simulink model "amon_model"  (R2025b)
settings: Solver=VariableStepAuto  StartTime=0.0  StopTime=dt  RelTol=1e-3
undefined symbols (not defined in the file or in its folder): EDF_max, EDF_min, g, servo1_offset, servo2_offset, servo3_offset, servo4_offset, servo_max, servo_min, tau_edf, tau_servo
libraries: simulink x1
settings Model: Creator=titit  LastModifiedBy=titit

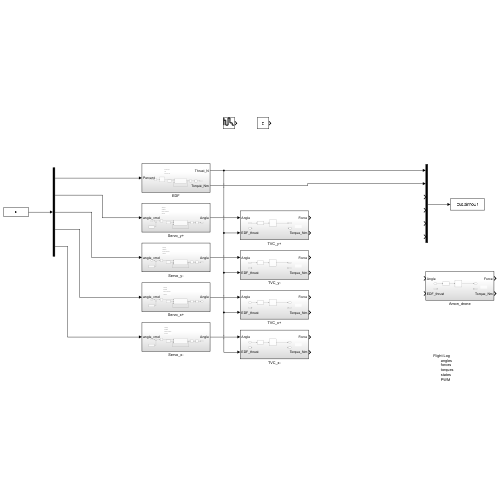
[thumbnail: Simulink's stored preview of the top-level diagram]
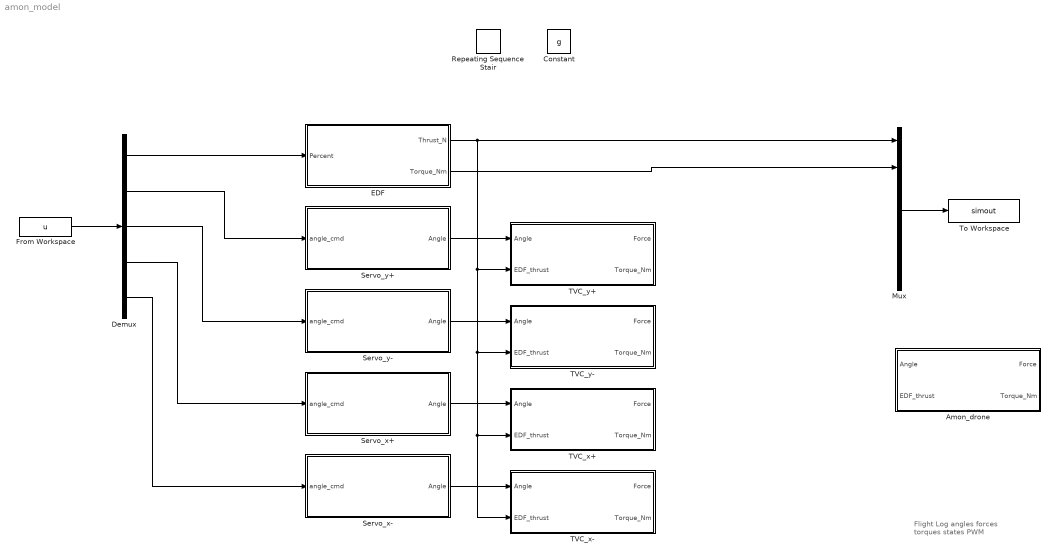
== system amon_model ==
  note: Flight Log
      | 	angles
      | 	forces
      | 	torques
      | 	states
      | 	PWM
  Amon_drone : Subsystem
  Constant : Constant  Value=g
  Demux : Demux  Outputs=5
  EDF : Subsystem
  From Workspace : FromWorkspace  VariableName=u
  Mux : Mux  Inputs=6
  Repeating Sequence Stair : simulink/Sources/Repeating Sequence Stair  OutValues=[3 1 4 2 1].'  tsamp=-1  OutMin=[]  OutMax=[]  OutDataTypeStr=double  OutputDataTypeScalingMode=double  OutDataType=fixdt(0,8)  ConRadixGroup=Best Precision: Vector-wise  OutScaling=2^-12
  Servo_x+ : Subsystem
  Servo_x- : Subsystem
  Servo_y+ : Subsystem
  Servo_y- : Subsystem
  TVC_x+ : Subsystem
  TVC_x- : Subsystem
  TVC_y+ : Subsystem
  TVC_y- : Subsystem
  To Workspace : ToWorkspace  VariableName=simout  SaveFormat=Timeseries  SampleTime=-1
  wires:
  From Workspace/1 -> Demux/1
  Mux/1 -> To Workspace/1
  EDF/1(Thrust_N) -> TVC_x-/2(EDF_thrust), TVC_x+/2(EDF_thrust), TVC_y-/2(EDF_thrust), TVC_y+/2(EDF_thrust), Mux/1
  EDF/2(Torque_Nm) -> Mux/2
  Servo_y+/1(Angle) -> TVC_y+/1(Angle)
  Servo_y-/1(Angle) -> TVC_y-/1(Angle)
  Servo_x+/1(Angle) -> TVC_x+/1(Angle)
  Servo_x-/1(Angle) -> TVC_x-/1(Angle)
  Demux/1 -> EDF/1(Percent)
  Demux/2 -> Servo_y+/1(angle_cmd)
  Demux/3 -> Servo_y-/1(angle_cmd)
  Demux/4 -> Servo_x+/1(angle_cmd)
  Demux/5 -> Servo_x-/1(angle_cmd)

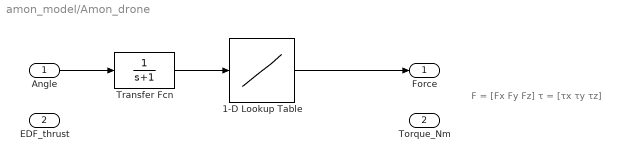
== system amon_model/Amon_drone ==
  note: F = [Fx Fy Fz]
      | τ = [τx τy τz]
  Angle : Inport
  EDF_thrust : Inport  Port=2
  1-D Lookup Table : Lookup_n-D  NumberOfTableDimensions=1  BreakpointsForDimension1=[-5:5]  Table=tanh([-5:5])  InternalRulePriority=Speed  RndMeth=Simplest
  Transfer Fcn : TransferFcn  Denominator=[1 1]
  Force : Outport
  Torque_Nm : Outport  Port=2
  wires:
  Transfer Fcn/1 -> 1-D Lookup Table/1
  Angle/1 -> Transfer Fcn/1
  1-D Lookup Table/1 -> Force/1

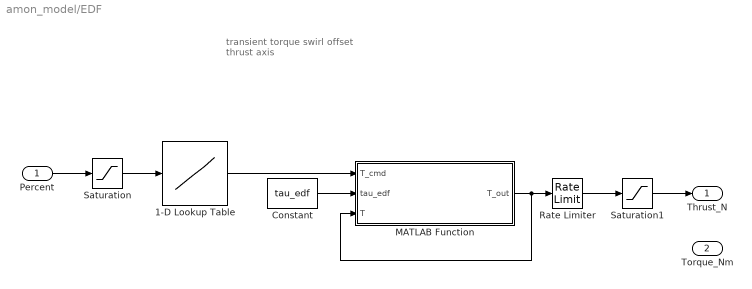
== system amon_model/EDF ==
  note: transient torque
      | swirl
      | offset thrust axis
  Percent : Inport
  1-D Lookup Table : Lookup_n-D  NumberOfTableDimensions=1  BreakpointsForDimension1=[-5:5]  Table=tanh([-5:5])  InternalRulePriority=Speed  RndMeth=Simplest
  Constant : Constant  Value=tau_edf
  MATLAB Function : MATLAB Function  TreatAsAtomicUnit=on
  Rate Limiter : RateLimiter  SampleTimeMode=inherited
  Saturation : Saturate  UpperLimit=EDF_max  LowerLimit=EDF_min
  Saturation1 : Saturate  UpperLimit=100  LowerLimit=0
  Thrust_N : Outport
  Torque_Nm : Outport  Port=2
  wires:
  Percent/1 -> Saturation/1
  Saturation1/1 -> Thrust_N/1
  1-D Lookup Table/1 -> MATLAB Function/1(T_cmd)
  MATLAB Function/1(T_out) -> MATLAB Function/3(T), Rate Limiter/1
  Saturation/1 -> 1-D Lookup Table/1
  Constant/1 -> MATLAB Function/2(tau_edf)
  Rate Limiter/1 -> Saturation1/1

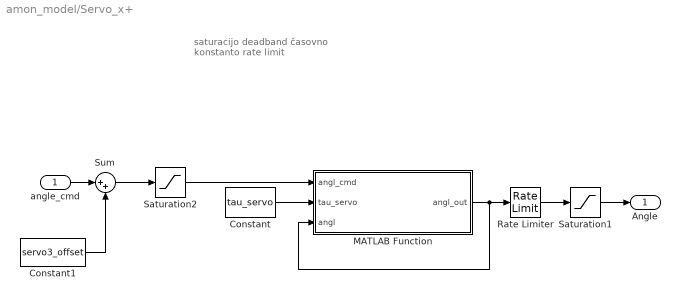
== system amon_model/Servo_x+ ==
  note: saturacijo
      | deadband
      | časovno konstanto
      | rate limit
  angle_cmd : Inport
  Constant : Constant  Value=tau_servo
  Constant1 : Constant  Value=servo3_offset
  MATLAB Function : MATLAB Function  TreatAsAtomicUnit=on
  Rate Limiter : RateLimiter  SampleTimeMode=inherited
  Saturation1 : Saturate  UpperLimit=servo_max  LowerLimit=servo_min
  Saturation2 : Saturate  UpperLimit=servo_max  LowerLimit=servo_min
  Sum : Sum  Inputs=|++
  Angle : Outport
  wires:
  Sum/1 -> Saturation2/1
  Constant/1 -> MATLAB Function/2(tau_servo)
  MATLAB Function/1(angl_out) -> Rate Limiter/1, MATLAB Function/3(angl)
  Saturation2/1 -> MATLAB Function/1(angl_cmd)
  Constant1/1 -> Sum/2
  angle_cmd/1 -> Sum/1
  Saturation1/1 -> Angle/1
  Rate Limiter/1 -> Saturation1/1

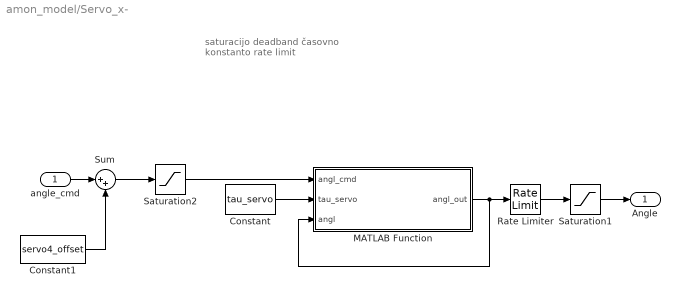
== system amon_model/Servo_x- ==
  note: saturacijo
      | deadband
      | časovno konstanto
      | rate limit
  angle_cmd : Inport
  Constant : Constant  Value=tau_servo
  Constant1 : Constant  Value=servo4_offset
  MATLAB Function : MATLAB Function  TreatAsAtomicUnit=on
  Rate Limiter : RateLimiter  SampleTimeMode=inherited
  Saturation1 : Saturate  UpperLimit=servo_max  LowerLimit=servo_min
  Saturation2 : Saturate  UpperLimit=servo_max  LowerLimit=servo_min
  Sum : Sum  Inputs=|++
  Angle : Outport
  wires:
  Constant/1 -> MATLAB Function/2(tau_servo)
  MATLAB Function/1(angl_out) -> Rate Limiter/1, MATLAB Function/3(angl)
  Saturation2/1 -> MATLAB Function/1(angl_cmd)
  Constant1/1 -> Sum/2
  angle_cmd/1 -> Sum/1
  Saturation1/1 -> Angle/1
  Rate Limiter/1 -> Saturation1/1
  Sum/1 -> Saturation2/1

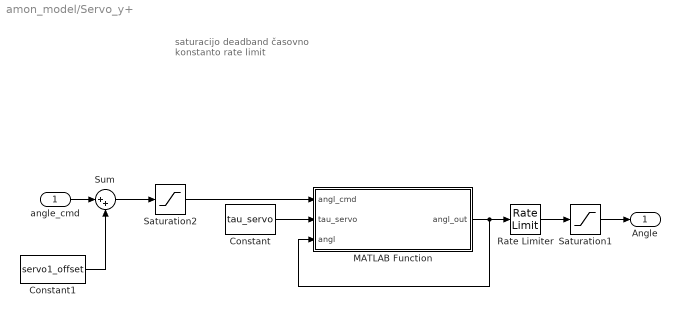
== system amon_model/Servo_y+ ==
  note: saturacijo
      | deadband
      | časovno konstanto
      | rate limit
  angle_cmd : Inport
  Constant : Constant  Value=tau_servo
  Constant1 : Constant  Value=servo1_offset
  MATLAB Function : MATLAB Function  TreatAsAtomicUnit=on
  Rate Limiter : RateLimiter  SampleTimeMode=inherited
  Saturation1 : Saturate  UpperLimit=servo_max  LowerLimit=servo_min
  Saturation2 : Saturate  UpperLimit=servo_max  LowerLimit=servo_min
  Sum : Sum  Inputs=|++
  Angle : Outport
  wires:
  Saturation2/1 -> MATLAB Function/1(angl_cmd)
  MATLAB Function/1(angl_out) -> MATLAB Function/3(angl), Rate Limiter/1
  Saturation1/1 -> Angle/1
  Constant/1 -> MATLAB Function/2(tau_servo)
  Rate Limiter/1 -> Saturation1/1
  angle_cmd/1 -> Sum/1
  Sum/1 -> Saturation2/1
  Constant1/1 -> Sum/2

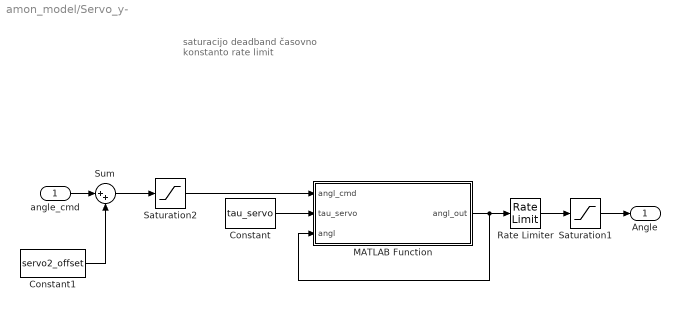
== system amon_model/Servo_y- ==
  note: saturacijo
      | deadband
      | časovno konstanto
      | rate limit
  angle_cmd : Inport
  Constant : Constant  Value=tau_servo
  Constant1 : Constant  Value=servo2_offset
  MATLAB Function : MATLAB Function  TreatAsAtomicUnit=on
  Rate Limiter : RateLimiter  SampleTimeMode=inherited
  Saturation1 : Saturate  UpperLimit=servo_max  LowerLimit=servo_min
  Saturation2 : Saturate  UpperLimit=servo_max  LowerLimit=servo_min
  Sum : Sum  Inputs=|++
  Angle : Outport
  wires:
  Sum/1 -> Saturation2/1
  Constant/1 -> MATLAB Function/2(tau_servo)
  MATLAB Function/1(angl_out) -> Rate Limiter/1, MATLAB Function/3(angl)
  Saturation2/1 -> MATLAB Function/1(angl_cmd)
  Constant1/1 -> Sum/2
  angle_cmd/1 -> Sum/1
  Saturation1/1 -> Angle/1
  Rate Limiter/1 -> Saturation1/1

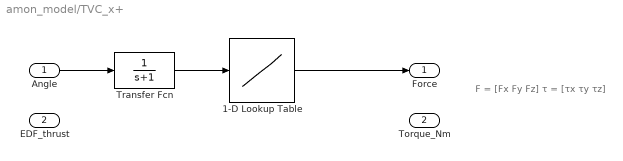
== system amon_model/TVC_x+ ==
  note: F = [Fx Fy Fz]
      | τ = [τx τy τz]
  Angle : Inport
  EDF_thrust : Inport  Port=2
  1-D Lookup Table : Lookup_n-D  NumberOfTableDimensions=1  BreakpointsForDimension1=[-5:5]  Table=tanh([-5:5])  InternalRulePriority=Speed  RndMeth=Simplest
  Transfer Fcn : TransferFcn  Denominator=[1 1]
  Force : Outport
  Torque_Nm : Outport  Port=2
  wires:
  Transfer Fcn/1 -> 1-D Lookup Table/1
  Angle/1 -> Transfer Fcn/1
  1-D Lookup Table/1 -> Force/1

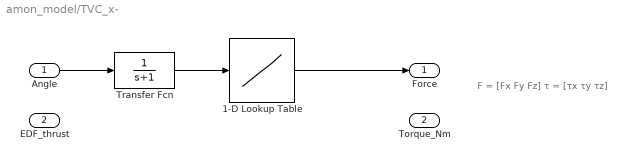
== system amon_model/TVC_x- ==
  note: F = [Fx Fy Fz]
      | τ = [τx τy τz]
  Angle : Inport
  EDF_thrust : Inport  Port=2
  1-D Lookup Table : Lookup_n-D  NumberOfTableDimensions=1  BreakpointsForDimension1=[-5:5]  Table=tanh([-5:5])  InternalRulePriority=Speed  RndMeth=Simplest
  Transfer Fcn : TransferFcn  Denominator=[1 1]
  Force : Outport
  Torque_Nm : Outport  Port=2
  wires:
  Transfer Fcn/1 -> 1-D Lookup Table/1
  Angle/1 -> Transfer Fcn/1
  1-D Lookup Table/1 -> Force/1

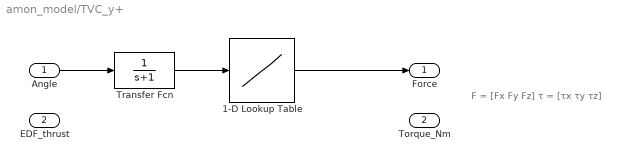
== system amon_model/TVC_y+ ==
  note: F = [Fx Fy Fz]
      | τ = [τx τy τz]
  Angle : Inport
  EDF_thrust : Inport  Port=2
  1-D Lookup Table : Lookup_n-D  NumberOfTableDimensions=1  BreakpointsForDimension1=[-5:5]  Table=tanh([-5:5])  InternalRulePriority=Speed  RndMeth=Simplest
  Transfer Fcn : TransferFcn  Denominator=[1 1]
  Force : Outport
  Torque_Nm : Outport  Port=2
  wires:
  Transfer Fcn/1 -> 1-D Lookup Table/1
  Angle/1 -> Transfer Fcn/1
  1-D Lookup Table/1 -> Force/1

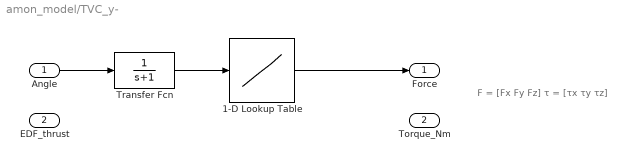
== system amon_model/TVC_y- ==
  note: F = [Fx Fy Fz]
      | τ = [τx τy τz]
  Angle : Inport
  EDF_thrust : Inport  Port=2
  1-D Lookup Table : Lookup_n-D  NumberOfTableDimensions=1  BreakpointsForDimension1=[-5:5]  Table=tanh([-5:5])  InternalRulePriority=Speed  RndMeth=Simplest
  Transfer Fcn : TransferFcn  Denominator=[1 1]
  Force : Outport
  Torque_Nm : Outport  Port=2
  wires:
  Transfer Fcn/1 -> 1-D Lookup Table/1
  Angle/1 -> Transfer Fcn/1
  1-D Lookup Table/1 -> Force/1

== matlab function amon_model/EDF/MATLAB Function ==
  data: T_cmd input; tau_edf input; T_out output; T input
function T_out = thrust_delay(T_cmd, tau_edf, T)
    T_out = (1/tau_edf) * (T_cmd - T);
end

== matlab function amon_model/Servo_y-/MATLAB Function ==
  data: angl_cmd input; tau_servo input; angl_out output; angl input
function angl_out = servo_delay(angl_cmd, tau_servo, angl)
    angl_out = (1/tau_servo) * (angl_cmd - angl);
end

== matlab function amon_model/Servo_x+/MATLAB Function ==
  data: angl_cmd input; tau_servo input; angl_out output; angl input
function angl_out = servo_delay(angl_cmd, tau_servo, angl)
    angl_out = (1/tau_servo) * (angl_cmd - angl);
end

== matlab function amon_model/Servo_x-/MATLAB Function ==
  data: angl_cmd input; tau_servo input; angl_out output; angl input
function angl_out = servo_delay(angl_cmd, tau_servo, angl)
    angl_out = (1/tau_servo) * (angl_cmd - angl);
end

== matlab function amon_model/Servo_y+/MATLAB Function ==
  data: angl_cmd input; tau_servo input; angl_out output; angl input
function angl_out = servo_delay(angl_cmd, tau_servo, angl)
    angl_out = (1/tau_servo) * (angl_cmd - angl);
end
